simulink library "halin"  (R2021b)
settings: Solver=VariableStepAuto  StartTime=0.0  StopTime=10.0  RelTol=1e-3
undefined symbols (not defined in the file): KHAL_CAN1ABM1E2E_flg, KHAL_CAN1EPB1E2E_flg, KHAL_CAN1EPS1E2E_flg, KHAL_CAN1ESC1E2E_flg, KHAL_CAN1ESC5E2E_flg, KHAL_CAN3BMS1E2E_flg, KHAL_CAN3BMS6E2E_flg, KHAL_CAN3CCU1E2E_flg, KHAL_CAN3CCU2E2E_flg, KHAL_CAN3MCUNF1E2E_flg, KHAL_CAN3MCUNR1E2E_flg, KHAL_CAN3Shifter1E2E_flg, KHAL_CAN3Shifter2E2E_flg, KHAL_CAN6FCM2E2E_flg, KHAL_CAN6FCM4E2E_flg, TRUE
libraries: simulink x645, FVT_lib x207, hcu_lib x59
(part 22 of 23)

== system halin/HAL_IN/CAN4/ZONE_FR_VCU/SOV2Err ==
  SOV2_Err : Inport
  UnitConverter : DataTypeConversion  OutDataTypeStr=uint8
  VHAL_SOV2Err_enum : Outport
  wires:
  UnitConverter/1 -> VHAL_SOV2Err_enum/1
  SOV2_Err/1 -> UnitConverter/1

== system halin/HAL_IN/CAN4/ZONE_FR_VCU/SOV3Err ==
  SOV3_Err : Inport
  UnitConverter : DataTypeConversion  OutDataTypeStr=uint8
  VHAL_SOV3Err_enum : Outport
  wires:
  UnitConverter/1 -> VHAL_SOV3Err_enum/1
  SOV3_Err/1 -> UnitConverter/1

== system halin/HAL_IN/CAN4/ZONE_FR_VCU/Tamb ==
  Tamb : Inport
  UnitConverter : DataTypeConversion  OutDataTypeStr=uint8
  convert_in : FVT_lib/hal/convert_in  gain=0.5  offset=-40
  VHAL_Tamb_C : Outport
  wires:
  convert_in/1 -> VHAL_Tamb_C/1
  UnitConverter/1 -> convert_in/1
  Tamb/1 -> UnitConverter/1

== system halin/HAL_IN/CAN4/ZONE_FR_VCU/TambErr ==
  Tamb_Err : Inport
  UnitConverter : DataTypeConversion  OutDataTypeStr=uint8
  VHAL_TambErr_enum : Outport
  wires:
  UnitConverter/1 -> VHAL_TambErr_enum/1
  Tamb_Err/1 -> UnitConverter/1

== system halin/HAL_IN/CAN4/zGW_APTC1/FrntPTCLeActHeatPwr ==
  FrntPTCLeActHeatPwr : Inport
  UnitConverter : DataTypeConversion  OutDataTypeStr=uint8
  convert_in : FVT_lib/hal/convert_in  gain=25  offset=0
  VHAL_FrntPTCLeActHeatPwr_W : Outport
  wires:
  convert_in/1 -> VHAL_FrntPTCLeActHeatPwr_W/1
  UnitConverter/1 -> convert_in/1
  FrntPTCLeActHeatPwr/1 -> UnitConverter/1

== system halin/HAL_IN/CAN4/zGW_APTC1/FrntPTCRearLeActHeatPwr ==
  FrntPTCRearLeActHeatPwr : Inport
  UnitConverter : DataTypeConversion  OutDataTypeStr=uint8
  convert_in : FVT_lib/hal/convert_in  gain=25  offset=0
  VHAL_FrntPTCRearLeActHeatPwr_W : Outport
  wires:
  convert_in/1 -> VHAL_FrntPTCRearLeActHeatPwr_W/1
  UnitConverter/1 -> convert_in/1
  FrntPTCRearLeActHeatPwr/1 -> UnitConverter/1

== system halin/HAL_IN/CAN4/zGW_APTC1/FrntPTCRearRiActHeatPwr ==
  FrntPTCRearRiActHeatPwr : Inport
  UnitConverter : DataTypeConversion  OutDataTypeStr=uint8
  convert_in : FVT_lib/hal/convert_in  gain=25  offset=0
  VHAL_FrntPTCRearRiActHeatPwr_W : Outport
  wires:
  convert_in/1 -> VHAL_FrntPTCRearRiActHeatPwr_W/1
  UnitConverter/1 -> convert_in/1
  FrntPTCRearRiActHeatPwr/1 -> UnitConverter/1

== system halin/HAL_IN/CAN4/zGW_APTC1/FrntPTCRiActHeatPwr ==
  FrntPTCRiActHeatPwr : Inport
  UnitConverter : DataTypeConversion  OutDataTypeStr=uint8
  convert_in : FVT_lib/hal/convert_in  gain=25  offset=0
  VHAL_FrntPTCRiActHeatPwr_W : Outport
  wires:
  convert_in/1 -> VHAL_FrntPTCRiActHeatPwr_W/1
  UnitConverter/1 -> convert_in/1
  FrntPTCRiActHeatPwr/1 -> UnitConverter/1

== system halin/HAL_IN/CAN4/zGW_CANFr1/COMPActualPwr ==
  COMP_ActualPwr : Inport
  UnitConverter : DataTypeConversion  OutDataTypeStr=uint16
  VHAL_COMPActualPwr_W : Outport
  wires:
  UnitConverter/1 -> VHAL_COMPActualPwr_W/1
  COMP_ActualPwr/1 -> UnitConverter/1

== system halin/HAL_IN/CAN4/zGW_CANFr1/COMPConCur ==
  COMP_ConCur : Inport
  UnitConverter : DataTypeConversion  OutDataTypeStr=uint16
  convert_in : FVT_lib/hal/convert_in  gain=0.02  offset=0
  VHAL_COMPConCur_A : Outport
  wires:
  convert_in/1 -> VHAL_COMPConCur_A/1
  UnitConverter/1 -> convert_in/1
  COMP_ConCur/1 -> UnitConverter/1

== system halin/HAL_IN/CAN4/zGW_CANFr1/COMPConVolt ==
  COMP_ConVolt : Inport
  UnitConverter : DataTypeConversion  OutDataTypeStr=uint16
  convert_in : FVT_lib/hal/convert_in  gain=0.02  offset=0
  VHAL_COMPConVolt_V : Outport
  wires:
  convert_in/1 -> VHAL_COMPConVolt_V/1
  UnitConverter/1 -> convert_in/1
  COMP_ConVolt/1 -> UnitConverter/1

== system halin/HAL_IN/CAN4/zGW_CANFr1/COMPStatorSpd ==
  COMP_StatorSpd : Inport
  UnitConverter : DataTypeConversion  OutDataTypeStr=uint16
  VHAL_COMPStatorSpd_rpm : Outport
  wires:
  UnitConverter/1 -> VHAL_COMPStatorSpd_rpm/1
  COMP_StatorSpd/1 -> UnitConverter/1

== system halin/HAL_IN/CAN4/zGW_CANFr1/PTC1PowerConsumption ==
  PTC1_PowerConsumption : Inport
  UnitConverter : DataTypeConversion  OutDataTypeStr=uint8
  convert_in : FVT_lib/hal/convert_in  gain=0.1  offset=0
  VHAL_PTC1PowerConsumption_kW : Outport
  wires:
  convert_in/1 -> VHAL_PTC1PowerConsumption_kW/1
  UnitConverter/1 -> convert_in/1
  PTC1_PowerConsumption/1 -> UnitConverter/1

== system halin/HAL_IN/CAN4/zGW_LINDr1/CSWDimSw ==
  CSW_DimSw : Inport
  UnitConverter : DataTypeConversion  OutDataTypeStr=uint8
  VHAL_CSWDimSw_flg : Outport
  wires:
  UnitConverter/1 -> VHAL_CSWDimSw_flg/1
  CSW_DimSw/1 -> UnitConverter/1

== system halin/HAL_IN/CAN4/zGW_LINDr1/CSWFWasSwSta ==
  CSW_FWasSw_Sta : Inport
  UnitConverter : DataTypeConversion  OutDataTypeStr=uint8
  VHAL_CSWFWasSwSta_enum : Outport
  wires:
  UnitConverter/1 -> VHAL_CSWFWasSwSta_enum/1
  CSW_FWasSw_Sta/1 -> UnitConverter/1

== system halin/HAL_IN/CAN4/zGW_LINDr1/CSWFWipSwSta ==
  CSW_FWipSw_Sta : Inport
  UnitConverter : DataTypeConversion  OutDataTypeStr=uint8
  VHAL_CSWFWipSwSta_enum : Outport
  wires:
  UnitConverter/1 -> VHAL_CSWFWipSwSta_enum/1
  CSW_FWipSw_Sta/1 -> UnitConverter/1

== system halin/HAL_IN/CAN4/zGW_LINDr1/CSWPassSWSta ==
  CSW_PassSW_Sta : Inport
  UnitConverter : DataTypeConversion  OutDataTypeStr=uint8
  VHAL_CSWPassSWSta_flg : Outport
  wires:
  UnitConverter/1 -> VHAL_CSWPassSWSta_flg/1
  CSW_PassSW_Sta/1 -> UnitConverter/1

== system halin/HAL_IN/CAN4/zGW_LINDr1/CSWRWasSWSta ==
  CSW_RWasSW_Sta : Inport
  UnitConverter : DataTypeConversion  OutDataTypeStr=uint8
  VHAL_CSWRWasSWSta_enum : Outport
  wires:
  UnitConverter/1 -> VHAL_CSWRWasSWSta_enum/1
  CSW_RWasSW_Sta/1 -> UnitConverter/1

== system halin/HAL_IN/CAN4/zGW_LINDr1/CSWRWipIntSwSta ==
  CSW_RWipIntSw_Sta : Inport
  UnitConverter : DataTypeConversion  OutDataTypeStr=uint8
  VHAL_CSWRWipIntSwSta_enum : Outport
  wires:
  UnitConverter/1 -> VHAL_CSWRWipIntSwSta_enum/1
  CSW_RWipIntSw_Sta/1 -> UnitConverter/1

== system halin/HAL_IN/CAN4/zGW_LINDr1/CSWTurnSwSta ==
  CSW_TurnSw_Sta : Inport
  UnitConverter : DataTypeConversion  OutDataTypeStr=uint8
  VHAL_CSWTurnSwSta_enum : Outport
  wires:
  UnitConverter/1 -> VHAL_CSWTurnSwSta_enum/1
  CSW_TurnSw_Sta/1 -> UnitConverter/1

== system halin/HAL_IN/CAN4/zGW_LINDr1/FAPWL01LINResponseError ==
  FAPWL_01_LIN_Response_Error : Inport
  UnitConverter : DataTypeConversion  OutDataTypeStr=uint8
  VHAL_FAPWL01LINResponseError_flg : Outport
  wires:
  UnitConverter/1 -> VHAL_FAPWL01LINResponseError_flg/1
  FAPWL_01_LIN_Response_Error/1 -> UnitConverter/1

== system halin/HAL_IN/CAN4/zGW_LINDr1/LDrvMotorRelayError ==
  L_Drv_Motor_Relay_Error : Inport
  UnitConverter : DataTypeConversion  OutDataTypeStr=uint8
  VHAL_LDrvMotorRelayError_flg : Outport
  wires:
  UnitConverter/1 -> VHAL_LDrvMotorRelayError_flg/1
  L_Drv_Motor_Relay_Error/1 -> UnitConverter/1

== system halin/HAL_IN/CAN4/zGW_LINDr1/LDrvMotorRippleError ==
  L_Drv_Motor_Ripple_Error : Inport
  UnitConverter : DataTypeConversion  OutDataTypeStr=uint8
  VHAL_LDrvMotorRippleError_flg : Outport
  wires:
  UnitConverter/1 -> VHAL_LDrvMotorRippleError_flg/1
  L_Drv_Motor_Ripple_Error/1 -> UnitConverter/1

== system halin/HAL_IN/CAN4/zGW_LINDr1/LDrvValWdwOpened ==
  L_Drv_Val_Wdw_Opened : Inport
  UnitConverter : DataTypeConversion  OutDataTypeStr=uint8
  VHAL_LDrvValWdwOpened_pct : Outport
  wires:
  UnitConverter/1 -> VHAL_LDrvValWdwOpened_pct/1
  L_Drv_Val_Wdw_Opened/1 -> UnitConverter/1

== system halin/HAL_IN/CAN4/zGW_LINDr1/LDrvWdwPositionSts ==
  L_Drv_Wdw_PositionSts : Inport
  UnitConverter : DataTypeConversion  OutDataTypeStr=uint8
  VHAL_LDrvWdwPositionSts_enum : Outport
  wires:
  UnitConverter/1 -> VHAL_LDrvWdwPositionSts_enum/1
  L_Drv_Wdw_PositionSts/1 -> UnitConverter/1

== system halin/HAL_IN/CAN4/zGW_LINDr1/LPasMotorRelayError ==
  L_Pas_Motor_Relay_Error : Inport
  UnitConverter : DataTypeConversion  OutDataTypeStr=uint8
  VHAL_LPasMotorRelayError_flg : Outport
  wires:
  UnitConverter/1 -> VHAL_LPasMotorRelayError_flg/1
  L_Pas_Motor_Relay_Error/1 -> UnitConverter/1

== system halin/HAL_IN/CAN4/zGW_LINDr1/LPasMotorRippleError ==
  L_Pas_Motor_Ripple_Error : Inport
  UnitConverter : DataTypeConversion  OutDataTypeStr=uint8
  VHAL_LPasMotorRippleError_flg : Outport
  wires:
  UnitConverter/1 -> VHAL_LPasMotorRippleError_flg/1
  L_Pas_Motor_Ripple_Error/1 -> UnitConverter/1

== system halin/HAL_IN/CAN4/zGW_LINDr1/LPasValWdwOpened ==
  L_Pas_Val_Wdw_Opened : Inport
  UnitConverter : DataTypeConversion  OutDataTypeStr=uint8
  VHAL_LPasValWdwOpened_pct : Outport
  wires:
  UnitConverter/1 -> VHAL_LPasValWdwOpened_pct/1
  L_Pas_Val_Wdw_Opened/1 -> UnitConverter/1

== system halin/HAL_IN/CAN4/zGW_LINDr1/LPasWdwPositionSts ==
  L_Pas_Wdw_PositionSts : Inport
  UnitConverter : DataTypeConversion  OutDataTypeStr=uint8
  VHAL_LPasWdwPositionSts_enum : Outport
  wires:
  UnitConverter/1 -> VHAL_LPasWdwPositionSts_enum/1
  L_Pas_Wdw_PositionSts/1 -> UnitConverter/1

== system halin/HAL_IN/CAN4/zGW_LINDr1/LRLDMotorRelayError ==
  L_RLD_Motor_Relay_Error : Inport
  UnitConverter : DataTypeConversion  OutDataTypeStr=uint8
  VHAL_LRLDMotorRelayError_flg : Outport
  wires:
  UnitConverter/1 -> VHAL_LRLDMotorRelayError_flg/1
  L_RLD_Motor_Relay_Error/1 -> UnitConverter/1

== system halin/HAL_IN/CAN4/zGW_LINDr1/LRLDMotorRippleError ==
  L_RLD_Motor_Ripple_Error : Inport
  UnitConverter : DataTypeConversion  OutDataTypeStr=uint8
  VHAL_LRLDMotorRippleError_flg : Outport
  wires:
  UnitConverter/1 -> VHAL_LRLDMotorRippleError_flg/1
  L_RLD_Motor_Ripple_Error/1 -> UnitConverter/1

== system halin/HAL_IN/CAN4/zGW_LINDr1/LRLDValWdwOpened ==
  L_RLD_Val_Wdw_Opened : Inport
  UnitConverter : DataTypeConversion  OutDataTypeStr=uint8
  VHAL_LRLDValWdwOpened_pct : Outport
  wires:
  UnitConverter/1 -> VHAL_LRLDValWdwOpened_pct/1
  L_RLD_Val_Wdw_Opened/1 -> UnitConverter/1

== system halin/HAL_IN/CAN4/zGW_LINDr1/LRLDWdwPositionSts ==
  L_RLD_Wdw_PositionSts : Inport
  UnitConverter : DataTypeConversion  OutDataTypeStr=uint8
  VHAL_LRLDWdwPositionSts_enum : Outport
  wires:
  UnitConverter/1 -> VHAL_LRLDWdwPositionSts_enum/1
  L_RLD_Wdw_PositionSts/1 -> UnitConverter/1

== system halin/HAL_IN/CAN4/zGW_LINDr1/LRRDMotorRelayError ==
  L_RRD_Motor_Relay_Error : Inport
  UnitConverter : DataTypeConversion  OutDataTypeStr=uint8
  VHAL_LRRDMotorRelayError_flg : Outport
  wires:
  UnitConverter/1 -> VHAL_LRRDMotorRelayError_flg/1
  L_RRD_Motor_Relay_Error/1 -> UnitConverter/1

== system halin/HAL_IN/CAN4/zGW_LINDr1/LRRDMotorRippleError ==
  L_RRD_Motor_Ripple_Error : Inport
  UnitConverter : DataTypeConversion  OutDataTypeStr=uint8
  VHAL_LRRDMotorRippleError_flg : Outport
  wires:
  UnitConverter/1 -> VHAL_LRRDMotorRippleError_flg/1
  L_RRD_Motor_Ripple_Error/1 -> UnitConverter/1

== system halin/HAL_IN/CAN4/zGW_LINDr1/LRRDValWdwOpened ==
  L_RRD_Val_Wdw_Opened : Inport
  UnitConverter : DataTypeConversion  OutDataTypeStr=uint8
  VHAL_LRRDValWdwOpened_pct : Outport
  wires:
  UnitConverter/1 -> VHAL_LRRDValWdwOpened_pct/1
  L_RRD_Val_Wdw_Opened/1 -> UnitConverter/1

== system halin/HAL_IN/CAN4/zGW_LINDr1/LRRDWdwPositionSts ==
  L_RRD_Wdw_PositionSts : Inport
  UnitConverter : DataTypeConversion  OutDataTypeStr=uint8
  VHAL_LRRDWdwPositionSts_enum : Outport
  wires:
  UnitConverter/1 -> VHAL_LRRDWdwPositionSts_enum/1
  L_RRD_Wdw_PositionSts/1 -> UnitConverter/1

== system halin/HAL_IN/CAN4/zGW_LINDr1/RAPWL01LINResponseError ==
  RAPWL_01_LIN_Response_Error : Inport
  UnitConverter : DataTypeConversion  OutDataTypeStr=uint8
  VHAL_RAPWL01LINResponseError_flg : Outport
  wires:
  UnitConverter/1 -> VHAL_RAPWL01LINResponseError_flg/1
  RAPWL_01_LIN_Response_Error/1 -> UnitConverter/1

== system halin/HAL_IN/CAN4/zGW_LINDr1/RLSLampSta ==
  RLS_Lamp_Sta : Inport
  UnitConverter : DataTypeConversion  OutDataTypeStr=uint8
  VHAL_RLSLampSta_flg : Outport
  wires:
  UnitConverter/1 -> VHAL_RLSLampSta_flg/1
  RLS_Lamp_Sta/1 -> UnitConverter/1

== system halin/HAL_IN/CAN4/zGW_LINDr1/RLSRainSnrWiperCmd ==
  RLS_RainSnrWiperCmd : Inport
  UnitConverter : DataTypeConversion  OutDataTypeStr=uint8
  VHAL_RLSRainSnrWiperCmd_enum : Outport
  wires:
  UnitConverter/1 -> VHAL_RLSRainSnrWiperCmd_enum/1
  RLS_RainSnrWiperCmd/1 -> UnitConverter/1

== system halin/HAL_IN/CAN4/zGW_LINDr1/SWC2LADASSta ==
  SWC2_L_ADAS_Sta : Inport
  UnitConverter : DataTypeConversion  OutDataTypeStr=uint8
  VHAL_SWC2LADASSta_flg : Outport
  wires:
  UnitConverter/1 -> VHAL_SWC2LADASSta_flg/1
  SWC2_L_ADAS_Sta/1 -> UnitConverter/1

== system halin/HAL_IN/CAN4/zGW_LINDr1/SWC2LDriveModeSta ==
  SWC2_L_DriveMode_Sta : Inport
  UnitConverter : DataTypeConversion  OutDataTypeStr=uint8
  VHAL_SWC2LDriveModeSta_flg : Outport
  wires:
  UnitConverter/1 -> VHAL_SWC2LDriveModeSta_flg/1
  SWC2_L_DriveMode_Sta/1 -> UnitConverter/1

== system halin/HAL_IN/CAN4/zGW_LINDr1/SWC2LHomeSta ==
  SWC2_L_Home_Sta : Inport
  UnitConverter : DataTypeConversion  OutDataTypeStr=uint8
  VHAL_SWC2LHomeSta_flg : Outport
  wires:
  UnitConverter/1 -> VHAL_SWC2LHomeSta_flg/1
  SWC2_L_Home_Sta/1 -> UnitConverter/1

== system halin/HAL_IN/CAN4/zGW_LINDr1/SWC2LLeftSta ==
  SWC2_L_Left_Sta : Inport
  UnitConverter : DataTypeConversion  OutDataTypeStr=uint8
  VHAL_SWC2LLeftSta_flg : Outport
  wires:
  UnitConverter/1 -> VHAL_SWC2LLeftSta_flg/1
  SWC2_L_Left_Sta/1 -> UnitConverter/1

== system halin/HAL_IN/CAN4/zGW_LINDr1/SWC2LRegenUpSta ==
  SWC2_L_RegenUp_Sta : Inport
  UnitConverter : DataTypeConversion  OutDataTypeStr=uint8
  VHAL_SWC2LRegenUpSta_flg : Outport
  wires:
  UnitConverter/1 -> VHAL_SWC2LRegenUpSta_flg/1
  SWC2_L_RegenUp_Sta/1 -> UnitConverter/1

== system halin/HAL_IN/CAN4/zGW_LINDr1/SWC2LRightSta ==
  SWC2_L_Right_Sta : Inport
  UnitConverter : DataTypeConversion  OutDataTypeStr=uint8
  VHAL_SWC2LRightSta_flg : Outport
  wires:
  UnitConverter/1 -> VHAL_SWC2LRightSta_flg/1
  SWC2_L_Right_Sta/1 -> UnitConverter/1

== system halin/HAL_IN/CAN4/zGW_LINDr1/SWC2LScrollDownSta ==
  SWC2_L_ScrollDown_Sta : Inport
  UnitConverter : DataTypeConversion  OutDataTypeStr=uint8
  VHAL_SWC2LScrollDownSta_flg : Outport
  wires:
  UnitConverter/1 -> VHAL_SWC2LScrollDownSta_flg/1
  SWC2_L_ScrollDown_Sta/1 -> UnitConverter/1

== system halin/HAL_IN/CAN4/zGW_LINDr1/SWC2LScrollPressSta ==
  SWC2_L_ScrollPress_Sta : Inport
  UnitConverter : DataTypeConversion  OutDataTypeStr=uint8
  VHAL_SWC2LScrollPressSta_flg : Outport
  wires:
  UnitConverter/1 -> VHAL_SWC2LScrollPressSta_flg/1
  SWC2_L_ScrollPress_Sta/1 -> UnitConverter/1

== system halin/HAL_IN/CAN4/zGW_LINDr1/SWC2LScrollUpSta ==
  SWC2_L_ScrollUp_Sta : Inport
  UnitConverter : DataTypeConversion  OutDataTypeStr=uint8
  VHAL_SWC2LScrollUpSta_flg : Outport
  wires:
  UnitConverter/1 -> VHAL_SWC2LScrollUpSta_flg/1
  SWC2_L_ScrollUp_Sta/1 -> UnitConverter/1

== system halin/HAL_IN/CAN4/zGW_LINDr1/SWC2RCustomizeSta ==
  SWC2_R_Customize_Sta : Inport
  UnitConverter : DataTypeConversion  OutDataTypeStr=uint8
  VHAL_SWC2RCustomizeSta_flg : Outport
  wires:
  UnitConverter/1 -> VHAL_SWC2RCustomizeSta_flg/1
  SWC2_R_Customize_Sta/1 -> UnitConverter/1

== system halin/HAL_IN/CAN4/zGW_LINDr1/SWC2RLeftSta ==
  SWC2_R_Left_Sta : Inport
  UnitConverter : DataTypeConversion  OutDataTypeStr=uint8
  VHAL_SWC2RLeftSta_flg : Outport
  wires:
  UnitConverter/1 -> VHAL_SWC2RLeftSta_flg/1
  SWC2_R_Left_Sta/1 -> UnitConverter/1

== system halin/HAL_IN/CAN4/zGW_LINDr1/SWC2RPageSwitchSta ==
  SWC2_R_PageSwitch_Sta : Inport
  UnitConverter : DataTypeConversion  OutDataTypeStr=uint8
  VHAL_SWC2RPageSwitchSta_flg : Outport
  wires:
  UnitConverter/1 -> VHAL_SWC2RPageSwitchSta_flg/1
  SWC2_R_PageSwitch_Sta/1 -> UnitConverter/1

== system halin/HAL_IN/CAN4/zGW_LINDr1/SWC2RRegenDownSta ==
  SWC2_R_RegenDown_Sta : Inport
  UnitConverter : DataTypeConversion  OutDataTypeStr=uint8
  VHAL_SWC2RRegenDownSta_flg : Outport
  wires:
  UnitConverter/1 -> VHAL_SWC2RRegenDownSta_flg/1
  SWC2_R_RegenDown_Sta/1 -> UnitConverter/1

== system halin/HAL_IN/CAN4/zGW_LINDr1/SWC2RRightSta ==
  SWC2_R_Right_Sta : Inport
  UnitConverter : DataTypeConversion  OutDataTypeStr=uint8
  VHAL_SWC2RRightSta_flg : Outport
  wires:
  UnitConverter/1 -> VHAL_SWC2RRightSta_flg/1
  SWC2_R_Right_Sta/1 -> UnitConverter/1

== system halin/HAL_IN/CAN4/zGW_LINDr1/SWC2RScrollDownSta ==
  SWC2_R_ScrollDown_Sta : Inport
  UnitConverter : DataTypeConversion  OutDataTypeStr=uint8
  VHAL_SWC2RScrollDownSta_flg : Outport
  wires:
  UnitConverter/1 -> VHAL_SWC2RScrollDownSta_flg/1
  SWC2_R_ScrollDown_Sta/1 -> UnitConverter/1

== system halin/HAL_IN/CAN4/zGW_LINDr1/SWC2RScrollPressSta ==
  SWC2_R_ScrollPress_Sta : Inport
  UnitConverter : DataTypeConversion  OutDataTypeStr=uint8
  VHAL_SWC2RScrollPressSta_flg : Outport
  wires:
  UnitConverter/1 -> VHAL_SWC2RScrollPressSta_flg/1
  SWC2_R_ScrollPress_Sta/1 -> UnitConverter/1

== system halin/HAL_IN/CAN4/zGW_LINDr1/SWC2RScrollUpSta ==
  SWC2_R_ScrollUp_Sta : Inport
  UnitConverter : DataTypeConversion  OutDataTypeStr=uint8
  VHAL_SWC2RScrollUpSta_flg : Outport
  wires:
  UnitConverter/1 -> VHAL_SWC2RScrollUpSta_flg/1
  SWC2_R_ScrollUp_Sta/1 -> UnitConverter/1

== system halin/HAL_IN/CAN4/zGW_LINDr1/SWC2RVRSta ==
  SWC2_R_VR_Sta : Inport
  UnitConverter : DataTypeConversion  OutDataTypeStr=uint8
  VHAL_SWC2RVRSta_flg : Outport
  wires:
  UnitConverter/1 -> VHAL_SWC2RVRSta_flg/1
  SWC2_R_VR_Sta/1 -> UnitConverter/1

== system halin/HAL_IN/CAN4/zGW_LINDr1/SWCACCSta ==
  SWC_ACC_Sta : Inport
  UnitConverter : DataTypeConversion  OutDataTypeStr=uint8
  VHAL_SWCACCSta_flg : Outport
  wires:
  UnitConverter/1 -> VHAL_SWCACCSta_flg/1
  SWC_ACC_Sta/1 -> UnitConverter/1

== system halin/HAL_IN/CAN4/zGW_LINDr1/SWCCANCELSta ==
  SWC_CANCEL_Sta : Inport
  UnitConverter : DataTypeConversion  OutDataTypeStr=uint8
  VHAL_SWCCANCELSta_flg : Outport
  wires:
  UnitConverter/1 -> VHAL_SWCCANCELSta_flg/1
  SWC_CANCEL_Sta/1 -> UnitConverter/1

== system halin/HAL_IN/CAN4/zGW_LINDr1/SWCDistanceSta ==
  SWC_Distance_Sta : Inport
  UnitConverter : DataTypeConversion  OutDataTypeStr=uint8
  VHAL_SWCDistanceSta_flg : Outport
  wires:
  UnitConverter/1 -> VHAL_SWCDistanceSta_flg/1
  SWC_Distance_Sta/1 -> UnitConverter/1

== system halin/HAL_IN/CAN4/zGW_LINDr1/SWCDownSta ==
  SWC_Down_Sta : Inport
  UnitConverter : DataTypeConversion  OutDataTypeStr=uint8
  VHAL_SWCDownSta_flg : Outport
  wires:
  UnitConverter/1 -> VHAL_SWCDownSta_flg/1
  SWC_Down_Sta/1 -> UnitConverter/1

== system halin/HAL_IN/CAN4/zGW_LINDr1/SWCLKASta ==
  SWC_LKA_Sta : Inport
  UnitConverter : DataTypeConversion  OutDataTypeStr=uint8
  VHAL_SWCLKASta_flg : Outport
  wires:
  UnitConverter/1 -> VHAL_SWCLKASta_flg/1
  SWC_LKA_Sta/1 -> UnitConverter/1

== system halin/HAL_IN/CAN4/zGW_LINDr1/SWCLeftSta ==
  SWC_Left_Sta : Inport
  UnitConverter : DataTypeConversion  OutDataTypeStr=uint8
  VHAL_SWCLeftSta_flg : Outport
  wires:
  UnitConverter/1 -> VHAL_SWCLeftSta_flg/1
  SWC_Left_Sta/1 -> UnitConverter/1

== system halin/HAL_IN/CAN4/zGW_LINDr1/SWCRegenDown ==
  SWC_RegenDown : Inport
  UnitConverter : DataTypeConversion  OutDataTypeStr=uint8
  VHAL_SWCRegenDown_flg : Outport
  wires:
  UnitConverter/1 -> VHAL_SWCRegenDown_flg/1
  SWC_RegenDown/1 -> UnitConverter/1

== system halin/HAL_IN/CAN4/zGW_LINDr1/SWCRegenUp ==
  SWC_RegenUp : Inport
  UnitConverter : DataTypeConversion  OutDataTypeStr=uint8
  VHAL_SWCRegenUp_flg : Outport
  wires:
  UnitConverter/1 -> VHAL_SWCRegenUp_flg/1
  SWC_RegenUp/1 -> UnitConverter/1

== system halin/HAL_IN/CAN4/zGW_LINDr1/SWCResUpSta ==
  SWC_Res_Up_Sta : Inport
  UnitConverter : DataTypeConversion  OutDataTypeStr=uint8
  VHAL_SWCResUpSta_flg : Outport
  wires:
  UnitConverter/1 -> VHAL_SWCResUpSta_flg/1
  SWC_Res_Up_Sta/1 -> UnitConverter/1

== system halin/HAL_IN/CAN4/zGW_LINDr1/SWCRightSta ==
  SWC_Right_Sta : Inport
  UnitConverter : DataTypeConversion  OutDataTypeStr=uint8
  VHAL_SWCRightSta_flg : Outport
  wires:
  UnitConverter/1 -> VHAL_SWCRightSta_flg/1
  SWC_Right_Sta/1 -> UnitConverter/1

== system halin/HAL_IN/CAN4/zGW_LINDr1/SWCSetdownSta ==
  SWC_Set_down_Sta : Inport
  UnitConverter : DataTypeConversion  OutDataTypeStr=uint8
  VHAL_SWCSetdownSta_flg : Outport
  wires:
  UnitConverter/1 -> VHAL_SWCSetdownSta_flg/1
  SWC_Set_down_Sta/1 -> UnitConverter/1

== system halin/HAL_IN/CAN4/zGW_LINDr1/SWCTripSta ==
  SWC_Trip_Sta : Inport
  UnitConverter : DataTypeConversion  OutDataTypeStr=uint8
  VHAL_SWCTripSta_flg : Outport
  wires:
  UnitConverter/1 -> VHAL_SWCTripSta_flg/1
  SWC_Trip_Sta/1 -> UnitConverter/1

== system halin/HAL_IN/CAN4/zGW_LINDr1/SWCUndefinedSta ==
  SWC_Undefined_Sta : Inport
  UnitConverter : DataTypeConversion  OutDataTypeStr=uint8
  VHAL_SWCUndefinedSta_flg : Outport
  wires:
  UnitConverter/1 -> VHAL_SWCUndefinedSta_flg/1
  SWC_Undefined_Sta/1 -> UnitConverter/1

== system halin/HAL_IN/CAN4/zGW_LINDr1/SWCUpSta ==
  SWC_Up_Sta : Inport
  UnitConverter : DataTypeConversion  OutDataTypeStr=uint8
  VHAL_SWCUpSta_flg : Outport
  wires:
  UnitConverter/1 -> VHAL_SWCUpSta_flg/1
  SWC_Up_Sta/1 -> UnitConverter/1

== system halin/HAL_IN/CAN4/zGW_LINDr1/SWCVRSta ==
  SWC_VR_Sta : Inport
  UnitConverter : DataTypeConversion  OutDataTypeStr=uint8
  VHAL_SWCVRSta_flg : Outport
  wires:
  UnitConverter/1 -> VHAL_SWCVRSta_flg/1
  SWC_VR_Sta/1 -> UnitConverter/1

== system halin/HAL_IN/CAN4/zGW_LINDr1/SWCmodeSta ==
  SWC_mode_Sta : Inport
  UnitConverter : DataTypeConversion  OutDataTypeStr=uint8
  VHAL_SWCmodeSta_flg : Outport
  wires:
  UnitConverter/1 -> VHAL_SWCmodeSta_flg/1
  SWC_mode_Sta/1 -> UnitConverter/1

== system halin/HAL_IN/CAN4/zGW_LINDr2/ACT1ResponseError ==
  ACT1_Response_Error : Inport
  UnitConverter : DataTypeConversion  OutDataTypeStr=uint8
  VHAL_ACT1ResponseError_flg : Outport
  wires:
  UnitConverter/1 -> VHAL_ACT1ResponseError_flg/1
  ACT1_Response_Error/1 -> UnitConverter/1

== system halin/HAL_IN/CAN4/zGW_LINFr1/AGSActualPosition ==
  AGS_Actual_Position : Inport
  UnitConverter : DataTypeConversion  OutDataTypeStr=uint8
  VHAL_AGSActualPosition_enum : Outport
  wires:
  UnitConverter/1 -> VHAL_AGSActualPosition_enum/1
  AGS_Actual_Position/1 -> UnitConverter/1

== system halin/HAL_IN/CAN4/zGW_LINFr1/FGSIntenRspSta ==
  FGS_IntenRsp_Sta : Inport
  UnitConverter : DataTypeConversion  OutDataTypeStr=uint8
  VHAL_FGSIntenRspSta_enum : Outport
  wires:
  UnitConverter/1 -> VHAL_FGSIntenRspSta_enum/1
  FGS_IntenRsp_Sta/1 -> UnitConverter/1

== system halin/HAL_IN/CAN4/zGW_LINFr2/EWP1BlockError ==
  EWP1_Block_Error : Inport
  UnitConverter : DataTypeConversion  OutDataTypeStr=uint8
  VHAL_EWP1BlockError_enum : Outport
  wires:
  UnitConverter/1 -> VHAL_EWP1BlockError_enum/1
  EWP1_Block_Error/1 -> UnitConverter/1

== system halin/HAL_IN/CAN4/zGW_LINFr2/EWP1OverCurrError ==
  EWP1_OverCurr_Error : Inport
  UnitConverter : DataTypeConversion  OutDataTypeStr=uint8
  VHAL_EWP1OverCurrError_enum : Outport
  wires:
  UnitConverter/1 -> VHAL_EWP1OverCurrError_enum/1
  EWP1_OverCurr_Error/1 -> UnitConverter/1

== system halin/HAL_IN/CAN4/zGW_LINFr2/EWP2BlockError ==
  EWP2_Block_Error : Inport
  UnitConverter : DataTypeConversion  OutDataTypeStr=uint8
  VHAL_EWP2BlockError_enum : Outport
  wires:
  UnitConverter/1 -> VHAL_EWP2BlockError_enum/1
  EWP2_Block_Error/1 -> UnitConverter/1

== system halin/HAL_IN/CAN4/zGW_LINFr2/EWP2OverCurrError ==
  EWP2_OverCurr_Error : Inport
  UnitConverter : DataTypeConversion  OutDataTypeStr=uint8
  VHAL_EWP2OverCurrError_enum : Outport
  wires:
  UnitConverter/1 -> VHAL_EWP2OverCurrError_enum/1
  EWP2_OverCurr_Error/1 -> UnitConverter/1

== system halin/HAL_IN/CAN4/zGW_LINFr2/EWP3BlockError ==
  EWP3_Block_Error : Inport
  UnitConverter : DataTypeConversion  OutDataTypeStr=uint8
  VHAL_EWP3BlockError_enum : Outport
  wires:
  UnitConverter/1 -> VHAL_EWP3BlockError_enum/1
  EWP3_Block_Error/1 -> UnitConverter/1

== system halin/HAL_IN/CAN4/zGW_LINFr2/EWP3OverCurrError ==
  EWP3_OverCurr_Error : Inport
  UnitConverter : DataTypeConversion  OutDataTypeStr=uint8
  VHAL_EWP3OverCurrError_enum : Outport
  wires:
  UnitConverter/1 -> VHAL_EWP3OverCurrError_enum/1
  EWP3_OverCurr_Error/1 -> UnitConverter/1

== system halin/HAL_IN/CAN4/zGW_SEAT1/DSEATAntiSta ==
  DSEAT_Anti_Sta : Inport
  UnitConverter : DataTypeConversion  OutDataTypeStr=uint8
  VHAL_DSEATAntiSta_flg : Outport
  wires:
  UnitConverter/1 -> VHAL_DSEATAntiSta_flg/1
  DSEAT_Anti_Sta/1 -> UnitConverter/1

== system halin/HAL_IN/CAN4/zGW_SEAT1/DSEATEntryFunSta ==
  DSEAT_EntryFun_Sta : Inport
  UnitConverter : DataTypeConversion  OutDataTypeStr=uint8
  VHAL_DSEATEntryFunSta_flg : Outport
  wires:
  UnitConverter/1 -> VHAL_DSEATEntryFunSta_flg/1
  DSEAT_EntryFun_Sta/1 -> UnitConverter/1

== system halin/HAL_IN/CAN4/zGW_SEAT1/DSEATErrorSta ==
  DSEAT_Error_Sta : Inport
  UnitConverter : DataTypeConversion  OutDataTypeStr=uint8
  VHAL_DSEATErrorSta_flg : Outport
  wires:
  UnitConverter/1 -> VHAL_DSEATErrorSta_flg/1
  DSEAT_Error_Sta/1 -> UnitConverter/1

== system halin/HAL_IN/CAN4/zGW_SEAT1/DSEATHWVer ==
  DSEAT_HW_Ver : Inport
  UnitConverter : DataTypeConversion  OutDataTypeStr=uint16
  VHAL_DSEATHWVer_enum : Outport
  wires:
  UnitConverter/1 -> VHAL_DSEATHWVer_enum/1
  DSEAT_HW_Ver/1 -> UnitConverter/1

== system halin/HAL_IN/CAN4/zGW_SEAT1/DSEATMode ==
  DSEAT_Mode : Inport
  UnitConverter : DataTypeConversion  OutDataTypeStr=uint8
  VHAL_DSEATMode_enum : Outport
  wires:
  UnitConverter/1 -> VHAL_DSEATMode_enum/1
  DSEAT_Mode/1 -> UnitConverter/1

== system halin/HAL_IN/CAN4/zGW_SEAT1/DSEATSWVer ==
  DSEAT_SW_Ver : Inport
  UnitConverter : DataTypeConversion  OutDataTypeStr=uint16
  VHAL_DSEATSWVer_enum : Outport
  wires:
  UnitConverter/1 -> VHAL_DSEATSWVer_enum/1
  DSEAT_SW_Ver/1 -> UnitConverter/1

== system halin/HAL_IN/CAN4/zGW_SEAT1/DSEATVentSta ==
  DSEAT_Vent_Sta : Inport
  UnitConverter : DataTypeConversion  OutDataTypeStr=uint8
  VHAL_DSEATVentSta_enum : Outport
  wires:
  UnitConverter/1 -> VHAL_DSEATVentSta_enum/1
  DSEAT_Vent_Sta/1 -> UnitConverter/1

== system halin/HAL_IN/CAN4/zGW_SEAT1/DSEATheatersta ==
  DSEAT_heater_sta : Inport
  UnitConverter : DataTypeConversion  OutDataTypeStr=uint8
  VHAL_DSEATheatersta_enum : Outport
  wires:
  UnitConverter/1 -> VHAL_DSEATheatersta_enum/1
  DSEAT_heater_sta/1 -> UnitConverter/1

== system halin/HAL_IN/CAN4/zGW_SEAT1/PSEATErrorSta ==
  PSEAT_Error_Sta : Inport
  UnitConverter : DataTypeConversion  OutDataTypeStr=uint8
  VHAL_PSEATErrorSta_flg : Outport
  wires:
  UnitConverter/1 -> VHAL_PSEATErrorSta_flg/1
  PSEAT_Error_Sta/1 -> UnitConverter/1

== system halin/HAL_IN/CAN4/zGW_SEAT1/PSEATHWVer ==
  PSEAT_HW_Ver : Inport
  UnitConverter : DataTypeConversion  OutDataTypeStr=uint16
  VHAL_PSEATHWVer_enum : Outport
  wires:
  UnitConverter/1 -> VHAL_PSEATHWVer_enum/1
  PSEAT_HW_Ver/1 -> UnitConverter/1

== system halin/HAL_IN/CAN4/zGW_SEAT1/PSEATMode ==
  PSEAT_Mode : Inport
  UnitConverter : DataTypeConversion  OutDataTypeStr=uint8
  VHAL_PSEATMode_enum : Outport
  wires:
  UnitConverter/1 -> VHAL_PSEATMode_enum/1
  PSEAT_Mode/1 -> UnitConverter/1

== system halin/HAL_IN/CAN4/zGW_SEAT1/PSEATSWVer ==
  PSEAT_SW_Ver : Inport
  UnitConverter : DataTypeConversion  OutDataTypeStr=uint16
  VHAL_PSEATSWVer_enum : Outport
  wires:
  UnitConverter/1 -> VHAL_PSEATSWVer_enum/1
  PSEAT_SW_Ver/1 -> UnitConverter/1

== system halin/HAL_IN/CAN4/zGW_SEAT1/PSEATVentSta ==
  PSEAT_Vent_Sta : Inport
  UnitConverter : DataTypeConversion  OutDataTypeStr=uint8
  VHAL_PSEATVentSta_enum : Outport
  wires:
  UnitConverter/1 -> VHAL_PSEATVentSta_enum/1
  PSEAT_Vent_Sta/1 -> UnitConverter/1

== system halin/HAL_IN/CAN4/zGW_SEAT1/PSEATheatersta ==
  PSEAT_heater_sta : Inport
  UnitConverter : DataTypeConversion  OutDataTypeStr=uint8
  VHAL_PSEATheatersta_enum : Outport
  wires:
  UnitConverter/1 -> VHAL_PSEATheatersta_enum/1
  PSEAT_heater_sta/1 -> UnitConverter/1

== system halin/HAL_IN/CAN6/FCM1/ACCComfortBandLower ==
  ACC_ComfortBandLower : Inport
  UnitConverter : DataTypeConversion  OutDataTypeStr=uint16
  convert_in : FVT_lib/hal/convert_in  gain=0.05  offset=-15
  VHAL_ACCComfortBandLower_mps2 : Outport
  wires:
  convert_in/1 -> VHAL_ACCComfortBandLower_mps2/1
  UnitConverter/1 -> convert_in/1
  ACC_ComfortBandLower/1 -> UnitConverter/1

== system halin/HAL_IN/CAN6/FCM1/ACCComfortBandUpper ==
  ACC_ComfortBandUpper : Inport
  UnitConverter : DataTypeConversion  OutDataTypeStr=uint16
  convert_in : FVT_lib/hal/convert_in  gain=0.05  offset=-15
  VHAL_ACCComfortBandUpper_mps2 : Outport
  wires:
  convert_in/1 -> VHAL_ACCComfortBandUpper_mps2/1
  UnitConverter/1 -> convert_in/1
  ACC_ComfortBandUpper/1 -> UnitConverter/1

== system halin/HAL_IN/CAN6/FCM1/ACCJerkLowerLimit ==
  ACC_JerkLowerLimit : Inport
  UnitConverter : DataTypeConversion  OutDataTypeStr=uint8
  convert_in : FVT_lib/hal/convert_in  gain=0.1  offset=-6
  VHAL_ACCJerkLowerLimit_mps3 : Outport
  wires:
  convert_in/1 -> VHAL_ACCJerkLowerLimit_mps3/1
  UnitConverter/1 -> convert_in/1
  ACC_JerkLowerLimit/1 -> UnitConverter/1

== system halin/HAL_IN/CAN6/FCM1/ACCJerkUpperLimit ==
  ACC_JerkUpperLimit : Inport
  UnitConverter : DataTypeConversion  OutDataTypeStr=uint8
  convert_in : FVT_lib/hal/convert_in  gain=0.1  offset=-6
  VHAL_ACCJerkUpperLimit_mps3 : Outport
  wires:
  convert_in/1 -> VHAL_ACCJerkUpperLimit_mps3/1
  UnitConverter/1 -> convert_in/1
  ACC_JerkUpperLimit/1 -> UnitConverter/1

== system halin/HAL_IN/CAN6/FCM1/ACCObjDist ==
  ACC_ObjDist : Inport
  UnitConverter : DataTypeConversion  OutDataTypeStr=uint16
  convert_in : FVT_lib/hal/convert_in  gain=0.1  offset=0
  VHAL_ACCObjDist_m : Outport
  wires:
  convert_in/1 -> VHAL_ACCObjDist_m/1
  UnitConverter/1 -> convert_in/1
  ACC_ObjDist/1 -> UnitConverter/1

== system halin/HAL_IN/CAN6/FCM1/ACCObjDstLvl ==
  ACC_ObjDstLvl : Inport
  UnitConverter : DataTypeConversion  OutDataTypeStr=uint8
  VHAL_ACCObjDstLvl_enum : Outport
  wires:
  UnitConverter/1 -> VHAL_ACCObjDstLvl_enum/1
  ACC_ObjDstLvl/1 -> UnitConverter/1

== system halin/HAL_IN/CAN6/FCM1/ACCObjRelSpd ==
  ACC_ObjRelSpd : Inport
  UnitConverter : DataTypeConversion  OutDataTypeStr=uint16
  convert_in : FVT_lib/hal/convert_in  gain=0.1  offset=-100
  VHAL_ACCObjRelSpd_mps : Outport
  wires:
  convert_in/1 -> VHAL_ACCObjRelSpd_mps/1
  UnitConverter/1 -> convert_in/1
  ACC_ObjRelSpd/1 -> UnitConverter/1

== system halin/HAL_IN/CAN6/FCM1/ACCRequiredAccel ==
  ACC_RequiredAccel : Inport
  UnitConverter : DataTypeConversion  OutDataTypeStr=uint16
  convert_in : FVT_lib/hal/convert_in  gain=0.05  offset=-15
  VHAL_ACCRequiredAccel_mps2 : Outport
  wires:
  convert_in/1 -> VHAL_ACCRequiredAccel_mps2/1
  UnitConverter/1 -> convert_in/1
  ACC_RequiredAccel/1 -> UnitConverter/1

== system halin/HAL_IN/CAN6/FCM1/ACCTakeoverReq ==
  ACC_TakeoverReq : Inport
  UnitConverter : DataTypeConversion  OutDataTypeStr=uint8
  VHAL_ACCTakeoverReq_flg : Outport
  wires:
  UnitConverter/1 -> VHAL_ACCTakeoverReq_flg/1
  ACC_TakeoverReq/1 -> UnitConverter/1

== system halin/HAL_IN/CAN6/FCM1/ACCVehHoldReq ==
  ACC_VehHoldReq : Inport
  UnitConverter : DataTypeConversion  OutDataTypeStr=uint8
  VHAL_ACCVehHoldReq_flg : Outport
  wires:
  UnitConverter/1 -> VHAL_ACCVehHoldReq_flg/1
  ACC_VehHoldReq/1 -> UnitConverter/1

== system halin/HAL_IN/CAN6/FCM1/ADASACCSta ==
  ADAS_ACC_Sta : Inport
  UnitConverter : DataTypeConversion  OutDataTypeStr=uint8
  VHAL_ADASACCSta_enum : Outport
  wires:
  UnitConverter/1 -> VHAL_ADASACCSta_enum/1
  ADAS_ACC_Sta/1 -> UnitConverter/1

== system halin/HAL_IN/CAN6/FCM1/ADASAEBReq ==
  ADAS_AEBReq : Inport
  UnitConverter : DataTypeConversion  OutDataTypeStr=uint8
  VHAL_ADASAEBReq_enum : Outport
  wires:
  UnitConverter/1 -> VHAL_ADASAEBReq_enum/1
  ADAS_AEBReq/1 -> UnitConverter/1

== system halin/HAL_IN/CAN6/FCM1/ADASAEBSta ==
  ADAS_AEB_Sta : Inport
  UnitConverter : DataTypeConversion  OutDataTypeStr=uint8
  VHAL_ADASAEBSta_enum : Outport
  wires:
  UnitConverter/1 -> VHAL_ADASAEBSta_enum/1
  ADAS_AEB_Sta/1 -> UnitConverter/1

== system halin/HAL_IN/CAN6/FCM1/ADASCAMSpdLim ==
  ADAS_CAM_SpdLim : Inport
  UnitConverter : DataTypeConversion  OutDataTypeStr=uint8
  VHAL_ADASCAMSpdLim_enum : Outport
  wires:
  UnitConverter/1 -> VHAL_ADASCAMSpdLim_enum/1
  ADAS_CAM_SpdLim/1 -> UnitConverter/1

== system halin/HAL_IN/CAN6/FCM1/ADASDBSReq ==
  ADAS_DBSReq : Inport
  UnitConverter : DataTypeConversion  OutDataTypeStr=uint8
  VHAL_ADASDBSReq_enum : Outport
  wires:
  UnitConverter/1 -> VHAL_ADASDBSReq_enum/1
  ADAS_DBSReq/1 -> UnitConverter/1

== system halin/HAL_IN/CAN6/FCM1/ADASFCWMute ==
  ADAS_FCW_Mute : Inport
  UnitConverter : DataTypeConversion  OutDataTypeStr=uint8
  VHAL_ADASFCWMute_flg : Outport
  wires:
  UnitConverter/1 -> VHAL_ADASFCWMute_flg/1
  ADAS_FCW_Mute/1 -> UnitConverter/1

== system halin/HAL_IN/CAN6/FCM1/ADASFCWSta ==
  ADAS_FCW_Sta : Inport
  UnitConverter : DataTypeConversion  OutDataTypeStr=uint8
  VHAL_ADASFCWSta_enum : Outport
  wires:
  UnitConverter/1 -> VHAL_ADASFCWSta_enum/1
  ADAS_FCW_Sta/1 -> UnitConverter/1

== system halin/HAL_IN/CAN6/FCM1/ADASFaultSta ==
  ADAS_FaultSta : Inport
  UnitConverter : DataTypeConversion  OutDataTypeStr=uint8
  VHAL_ADASFaultSta_flg : Outport
  wires:
  UnitConverter/1 -> VHAL_ADASFaultSta_flg/1
  ADAS_FaultSta/1 -> UnitConverter/1

== system halin/HAL_IN/CAN6/FCM1/ADASFltWrnReq ==
  ADAS_FltWrnReq : Inport
  UnitConverter : DataTypeConversion  OutDataTypeStr=uint8
  VHAL_ADASFltWrnReq_flg : Outport
  wires:
  UnitConverter/1 -> VHAL_ADASFltWrnReq_flg/1
  ADAS_FltWrnReq/1 -> UnitConverter/1

== system halin/HAL_IN/CAN6/FCM1/ADASForceIdle ==
  ADAS_ForceIdle : Inport
  UnitConverter : DataTypeConversion  OutDataTypeStr=uint8
  VHAL_ADASForceIdle_flg : Outport
  wires:
  UnitConverter/1 -> VHAL_ADASForceIdle_flg/1
  ADAS_ForceIdle/1 -> UnitConverter/1

== system halin/HAL_IN/CAN6/FCM1/ADASISASta ==
  ADAS_ISA_Sta : Inport
  UnitConverter : DataTypeConversion  OutDataTypeStr=uint8
  VHAL_ADASISASta_enum : Outport
  wires:
  UnitConverter/1 -> VHAL_ADASISASta_enum/1
  ADAS_ISA_Sta/1 -> UnitConverter/1

== system halin/HAL_IN/CAN6/FCM1/ADASLDWMute ==
  ADAS_LDW_Mute : Inport
  UnitConverter : DataTypeConversion  OutDataTypeStr=uint8
  VHAL_ADASLDWMute_flg : Outport
  wires:
  UnitConverter/1 -> VHAL_ADASLDWMute_flg/1
  ADAS_LDW_Mute/1 -> UnitConverter/1

== system halin/HAL_IN/CAN6/FCM1/ADASLDWSta ==
  ADAS_LDW_Sta : Inport
  UnitConverter : DataTypeConversion  OutDataTypeStr=uint8
  VHAL_ADASLDWSta_enum : Outport
  wires:
  UnitConverter/1 -> VHAL_ADASLDWSta_enum/1
  ADAS_LDW_Sta/1 -> UnitConverter/1

== system halin/HAL_IN/CAN6/FCM1/ADASLFCHandsOffWarning ==
  ADAS_LFC_Hands_Off_Warning : Inport
  UnitConverter : DataTypeConversion  OutDataTypeStr=uint8
  VHAL_ADASLFCHandsOffWarning_enum : Outport
  wires:
  UnitConverter/1 -> VHAL_ADASLFCHandsOffWarning_enum/1
  ADAS_LFC_Hands_Off_Warning/1 -> UnitConverter/1

== system halin/HAL_IN/CAN6/FCM1/ADASLFCSta ==
  ADAS_LFC_Sta : Inport
  UnitConverter : DataTypeConversion  OutDataTypeStr=uint8
  VHAL_ADASLFCSta_enum : Outport
  wires:
  UnitConverter/1 -> VHAL_ADASLFCSta_enum/1
  ADAS_LFC_Sta/1 -> UnitConverter/1

== system halin/HAL_IN/CAN6/FCM1/ADASLFCWarnSound ==
  ADAS_LFC_Warn_Sound : Inport
  UnitConverter : DataTypeConversion  OutDataTypeStr=uint16
  VHAL_ADASLFCWarnSound_enum : Outport
  wires:
  UnitConverter/1 -> VHAL_ADASLFCWarnSound_enum/1
  ADAS_LFC_Warn_Sound/1 -> UnitConverter/1

== system halin/HAL_IN/CAN6/FCM1/ADASLKASta ==
  ADAS_LKA_Sta : Inport
  UnitConverter : DataTypeConversion  OutDataTypeStr=uint16
  VHAL_ADASLKASta_enum : Outport
  wires:
  UnitConverter/1 -> VHAL_ADASLKASta_enum/1
  ADAS_LKA_Sta/1 -> UnitConverter/1

== system halin/HAL_IN/CAN6/FCM1/ADASLaneModeL ==
  ADAS_LaneModeL : Inport
  UnitConverter : DataTypeConversion  OutDataTypeStr=uint16
  VHAL_ADASLaneModeL_enum : Outport
  wires:
  UnitConverter/1 -> VHAL_ADASLaneModeL_enum/1
  ADAS_LaneModeL/1 -> UnitConverter/1

== system halin/HAL_IN/CAN6/FCM1/ADASLaneModeR ==
  ADAS_LaneModeR : Inport
  UnitConverter : DataTypeConversion  OutDataTypeStr=uint8
  VHAL_ADASLaneModeR_enum : Outport
  wires:
  UnitConverter/1 -> VHAL_ADASLaneModeR_enum/1
  ADAS_LaneModeR/1 -> UnitConverter/1

== system halin/HAL_IN/CAN6/FCM1/ADASLanecurveL ==
  ADAS_Lane_curveL : Inport
  UnitConverter : DataTypeConversion  OutDataTypeStr=uint8
  convert_in : FVT_lib/hal/convert_in  gain=0.0005  offset=-0.03
  VHAL_ADASLanecurveL_raw32 : Outport
  wires:
  convert_in/1 -> VHAL_ADASLanecurveL_raw32/1
  UnitConverter/1 -> convert_in/1
  ADAS_Lane_curveL/1 -> UnitConverter/1

== system halin/HAL_IN/CAN6/FCM1/ADASLanecurveR ==
  ADAS_Lane_curveR : Inport
  UnitConverter : DataTypeConversion  OutDataTypeStr=uint8
  convert_in : FVT_lib/hal/convert_in  gain=0.0005  offset=-0.03
  VHAL_ADASLanecurveR_raw32 : Outport
  wires:
  convert_in/1 -> VHAL_ADASLanecurveR_raw32/1
  UnitConverter/1 -> convert_in/1
  ADAS_Lane_curveR/1 -> UnitConverter/1

== system halin/HAL_IN/CAN6/FCM1/ADASLanetypeL ==
  ADAS_LanetypeL : Inport
  UnitConverter : DataTypeConversion  OutDataTypeStr=uint16
  VHAL_ADASLanetypeL_enum : Outport
  wires:
  UnitConverter/1 -> VHAL_ADASLanetypeL_enum/1
  ADAS_LanetypeL/1 -> UnitConverter/1

== system halin/HAL_IN/CAN6/FCM1/ADASLanetypeR ==
  ADAS_LanetypeR : Inport
  UnitConverter : DataTypeConversion  OutDataTypeStr=uint8
  VHAL_ADASLanetypeR_enum : Outport
  wires:
  UnitConverter/1 -> VHAL_ADASLanetypeR_enum/1
  ADAS_LanetypeR/1 -> UnitConverter/1

== system halin/HAL_IN/CAN6/FCM1/ADASSLIFSpdLim ==
  ADAS_SLIF_SpdLim : Inport
  UnitConverter : DataTypeConversion  OutDataTypeStr=uint8
  VHAL_ADASSLIFSpdLim_enum : Outport
  wires:
  UnitConverter/1 -> VHAL_ADASSLIFSpdLim_enum/1
  ADAS_SLIF_SpdLim/1 -> UnitConverter/1

== system halin/HAL_IN/CAN6/FCM1/ADASSLIFSta ==
  ADAS_SLIF_Sta : Inport
  UnitConverter : DataTypeConversion  OutDataTypeStr=uint8
  VHAL_ADASSLIFSta_enum : Outport
  wires:
  UnitConverter/1 -> VHAL_ADASSLIFSta_enum/1
  ADAS_SLIF_Sta/1 -> UnitConverter/1

== system halin/HAL_IN/CAN6/FCM1/ADASShftPosnReq ==
  ADAS_ShftPosnReq : Inport
  UnitConverter : DataTypeConversion  OutDataTypeStr=uint8
  VHAL_ADASShftPosnReq_enum : Outport
  wires:
  UnitConverter/1 -> VHAL_ADASShftPosnReq_enum/1
  ADAS_ShftPosnReq/1 -> UnitConverter/1

== system halin/HAL_IN/CAN6/FCM1/ADASShftPosnReqA ==
  ADAS_ShftPosnReq_A : Inport
  UnitConverter : DataTypeConversion  OutDataTypeStr=uint8
  VHAL_ADASShftPosnReqA_flg : Outport
  wires:
  UnitConverter/1 -> VHAL_ADASShftPosnReqA_flg/1
  ADAS_ShftPosnReq_A/1 -> UnitConverter/1

== system halin/HAL_IN/CAN6/FCM1/ADASVehSpdLim ==
  ADAS_VehSpdLim : Inport
  UnitConverter : DataTypeConversion  OutDataTypeStr=uint8
  VHAL_ADASVehSpdLim_enum : Outport
  wires:
  UnitConverter/1 -> VHAL_ADASVehSpdLim_enum/1
  ADAS_VehSpdLim/1 -> UnitConverter/1

== system halin/HAL_IN/CAN6/FCM1/ADASWarningMsg ==
  ADAS_WarningMsg : Inport
  UnitConverter : DataTypeConversion  OutDataTypeStr=uint8
  VHAL_ADASWarningMsg_enum : Outport
  wires:
  UnitConverter/1 -> VHAL_ADASWarningMsg_enum/1
  ADAS_WarningMsg/1 -> UnitConverter/1

== system halin/HAL_IN/CAN6/FCM1/AEBVehHoldReq ==
  AEB_VehHoldReq : Inport
  UnitConverter : DataTypeConversion  OutDataTypeStr=uint8
  VHAL_AEBVehHoldReq_flg : Outport
  wires:
  UnitConverter/1 -> VHAL_AEBVehHoldReq_flg/1
  AEB_VehHoldReq/1 -> UnitConverter/1

== system halin/HAL_IN/CAN6/FCM1/CameraBlockage ==
  CameraBlockage : Inport
  UnitConverter : DataTypeConversion  OutDataTypeStr=uint8
  VHAL_CameraBlockage_flg : Outport
  wires:
  UnitConverter/1 -> VHAL_CameraBlockage_flg/1
  CameraBlockage/1 -> UnitConverter/1

== system halin/HAL_IN/CAN6/FCM1/FCM1Checksum ==
  FCM1_Checksum : Inport
  UnitConverter : DataTypeConversion  OutDataTypeStr=uint8
  VHAL_FCM1Checksum_enum : Outport
  wires:
  UnitConverter/1 -> VHAL_FCM1Checksum_enum/1
  FCM1_Checksum/1 -> UnitConverter/1

== system halin/HAL_IN/CAN6/FCM1/FCM1LifeCount ==
  FCM1_LifeCount : Inport
  UnitConverter : DataTypeConversion  OutDataTypeStr=uint8
  VHAL_FCM1LifeCount_enum : Outport
  wires:
  UnitConverter/1 -> VHAL_FCM1LifeCount_enum/1
  FCM1_LifeCount/1 -> UnitConverter/1

== system halin/HAL_IN/CAN6/FCM1/FCMACCmode ==
  FCM_ACCmode : Inport
  UnitConverter : DataTypeConversion  OutDataTypeStr=uint8
  VHAL_FCMACCmode_enum : Outport
  wires:
  UnitConverter/1 -> VHAL_FCMACCmode_enum/1
  FCM_ACCmode/1 -> UnitConverter/1

== system halin/HAL_IN/CAN6/FCM1/FCMLKAStrToqReq ==
  FCM_LKA_StrToqReq : Inport
  UnitConverter : DataTypeConversion  OutDataTypeStr=uint16
  convert_in : FVT_lib/hal/convert_in  gain=0.008  offset=-8
  VHAL_FCMLKAStrToqReq_Nm : Outport
  wires:
  convert_in/1 -> VHAL_FCMLKAStrToqReq_Nm/1
  UnitConverter/1 -> convert_in/1
  FCM_LKA_StrToqReq/1 -> UnitConverter/1

== system halin/HAL_IN/CAN6/FCM1/FCMLKATOIAct ==
  FCM_LKA_TOIAct : Inport
  UnitConverter : DataTypeConversion  OutDataTypeStr=uint8
  VHAL_FCMLKATOIAct_enum : Outport
  wires:
  UnitConverter/1 -> VHAL_FCMLKATOIAct_enum/1
  FCM_LKA_TOIAct/1 -> UnitConverter/1

== system halin/HAL_IN/CAN6/FCM1/FCMLKATOIFault ==
  FCM_LKA_TOIFault : Inport
  UnitConverter : DataTypeConversion  OutDataTypeStr=uint8
  VHAL_FCMLKATOIFault_flg : Outport
  wires:
  UnitConverter/1 -> VHAL_FCMLKATOIFault_flg/1
  FCM_LKA_TOIFault/1 -> UnitConverter/1

== system halin/HAL_IN/CAN6/FCM1/ForceLowBeam ==
  ForceLowBeam : Inport
  UnitConverter : DataTypeConversion  OutDataTypeStr=uint8
  VHAL_ForceLowBeam_enum : Outport
  wires:
  UnitConverter/1 -> VHAL_ForceLowBeam_enum/1
  ForceLowBeam/1 -> UnitConverter/1

== system halin/HAL_IN/CAN6/FCM1/HazardWarningReq ==
  HazardWarningReq : Inport
  UnitConverter : DataTypeConversion  OutDataTypeStr=uint8
  VHAL_HazardWarningReq_flg : Outport
  wires:
  UnitConverter/1 -> VHAL_HazardWarningReq_flg/1
  HazardWarningReq/1 -> UnitConverter/1

== system halin/HAL_IN/CAN6/FCM1/ISAWarningMsg ==
  ISA_WarningMsg : Inport
  UnitConverter : DataTypeConversion  OutDataTypeStr=uint8
  VHAL_ISAWarningMsg_enum : Outport
  wires:
  UnitConverter/1 -> VHAL_ISAWarningMsg_enum/1
  ISA_WarningMsg/1 -> UnitConverter/1

== system halin/HAL_IN/CAN6/FCM1/LKAHODDisplayWarning ==
  LKA_HOD_Display_Warning : Inport
  UnitConverter : DataTypeConversion  OutDataTypeStr=uint8
  VHAL_LKAHODDisplayWarning_flg : Outport
  wires:
  UnitConverter/1 -> VHAL_LKAHODDisplayWarning_flg/1
  LKA_HOD_Display_Warning/1 -> UnitConverter/1

== system halin/HAL_IN/CAN6/FCM1/LKAHODSoundWarning ==
  LKA_HOD_Sound_Warning : Inport
  UnitConverter : DataTypeConversion  OutDataTypeStr=uint8
  VHAL_LKAHODSoundWarning_flg : Outport
  wires:
  UnitConverter/1 -> VHAL_LKAHODSoundWarning_flg/1
  LKA_HOD_Sound_Warning/1 -> UnitConverter/1

== system halin/HAL_IN/CAN6/FCM1/LVDAACCStatusInformation ==
  LVDA_ACCStatusInformation : Inport
  UnitConverter : DataTypeConversion  OutDataTypeStr=uint8
  VHAL_LVDAACCStatusInformation_flg : Outport
  wires:
  UnitConverter/1 -> VHAL_LVDAACCStatusInformation_flg/1
  LVDA_ACCStatusInformation/1 -> UnitConverter/1

== system halin/HAL_IN/CAN6/FCM1/LVDADisabled ==
  LVDA_Disabled : Inport
  UnitConverter : DataTypeConversion  OutDataTypeStr=uint8
  VHAL_LVDADisabled_flg : Outport
  wires:
  UnitConverter/1 -> VHAL_LVDADisabled_flg/1
  LVDA_Disabled/1 -> UnitConverter/1

== system halin/HAL_IN/CAN6/FCM1/LVDAFailinfo ==
  LVDA_Failinfo : Inport
  UnitConverter : DataTypeConversion  OutDataTypeStr=uint8
  VHAL_LVDAFailinfo_flg : Outport
  wires:
  UnitConverter/1 -> VHAL_LVDAFailinfo_flg/1
  LVDA_Failinfo/1 -> UnitConverter/1

== system halin/HAL_IN/CAN6/FCM1/LVDAMuteSta ==
  LVDA_Mute_Sta : Inport
  UnitConverter : DataTypeConversion  OutDataTypeStr=uint8
  VHAL_LVDAMuteSta_enum : Outport
  wires:
  UnitConverter/1 -> VHAL_LVDAMuteSta_enum/1
  LVDA_Mute_Sta/1 -> UnitConverter/1

== system halin/HAL_IN/CAN6/FCM1/LVDAWarning ==
  LVDA_Warning : Inport
  UnitConverter : DataTypeConversion  OutDataTypeStr=uint8
  VHAL_LVDAWarning_flg : Outport
  wires:
  UnitConverter/1 -> VHAL_LVDAWarning_flg/1
  LVDA_Warning/1 -> UnitConverter/1

== system halin/HAL_IN/CAN6/FCM1/LeftTurnLightReq ==
  LeftTurnLightReq : Inport
  UnitConverter : DataTypeConversion  OutDataTypeStr=uint8
  VHAL_LeftTurnLightReq_flg : Outport
  wires:
  UnitConverter/1 -> VHAL_LeftTurnLightReq_flg/1
  LeftTurnLightReq/1 -> UnitConverter/1

== system halin/HAL_IN/CAN6/FCM1/RightTurnLightReq ==
  RightTurnLightReq : Inport
  UnitConverter : DataTypeConversion  OutDataTypeStr=uint8
  VHAL_RightTurnLightReq_flg : Outport
  wires:
  UnitConverter/1 -> VHAL_RightTurnLightReq_flg/1
  RightTurnLightReq/1 -> UnitConverter/1

== system halin/HAL_IN/CAN6/FCM1/TargetType ==
  Target_Type : Inport
  UnitConverter : DataTypeConversion  OutDataTypeStr=uint16
  VHAL_TargetType_enum : Outport
  wires:
  UnitConverter/1 -> VHAL_TargetType_enum/1
  Target_Type/1 -> UnitConverter/1

== system halin/HAL_IN/CAN6/FCM1/TimeGapLevel ==
  TimeGapLevel : Inport
  UnitConverter : DataTypeConversion  OutDataTypeStr=uint8
  VHAL_TimeGapLevel_enum : Outport
  wires:
  UnitConverter/1 -> VHAL_TimeGapLevel_enum/1
  TimeGapLevel/1 -> UnitConverter/1

== system halin/HAL_IN/CAN6/FCM2/ADBVehDst1Val ==
  ADB_VehDst1Val : Inport
  UnitConverter : DataTypeConversion  OutDataTypeStr=uint8
  VHAL_ADBVehDst1Val_enum : Outport
  wires:
  UnitConverter/1 -> VHAL_ADBVehDst1Val_enum/1
  ADB_VehDst1Val/1 -> UnitConverter/1

== system halin/HAL_IN/CAN6/FCM3/MELaneCurvDervLt ==
  ME_Lane_CurvDervLt : Inport
  UnitConverter : DataTypeConversion  OutDataTypeStr=uint16
  convert_in : FVT_lib/hal/convert_in  gain=4e-09  offset=-0.00013
  VHAL_MELaneCurvDervLt_raw32 : Outport
  wires:
  convert_in/1 -> VHAL_MELaneCurvDervLt_raw32/1
  UnitConverter/1 -> convert_in/1
  ME_Lane_CurvDervLt/1 -> UnitConverter/1

== system halin/HAL_IN/CAN6/FCM3/MELaneCurvDervLt2 ==
  ME_Lane_CurvDervLt2 : Inport
  UnitConverter : DataTypeConversion  OutDataTypeStr=uint16
  convert_in : FVT_lib/hal/convert_in  gain=4e-09  offset=-0.00013
  VHAL_MELaneCurvDervLt2_raw32 : Outport
  wires:
  convert_in/1 -> VHAL_MELaneCurvDervLt2_raw32/1
  UnitConverter/1 -> convert_in/1
  ME_Lane_CurvDervLt2/1 -> UnitConverter/1

== system halin/HAL_IN/CAN6/FCM3/MELaneCurvDervRt ==
  ME_Lane_CurvDervRt : Inport
  UnitConverter : DataTypeConversion  OutDataTypeStr=uint16
  convert_in : FVT_lib/hal/convert_in  gain=4e-09  offset=-0.00013
  VHAL_MELaneCurvDervRt_raw32 : Outport
  wires:
  convert_in/1 -> VHAL_MELaneCurvDervRt_raw32/1
  UnitConverter/1 -> convert_in/1
  ME_Lane_CurvDervRt/1 -> UnitConverter/1

== system halin/HAL_IN/CAN6/FCM3/MELaneCurvDervRt2 ==
  ME_Lane_CurvDervRt2 : Inport
  UnitConverter : DataTypeConversion  OutDataTypeStr=uint16
  convert_in : FVT_lib/hal/convert_in  gain=4e-09  offset=-0.00013
  VHAL_MELaneCurvDervRt2_raw32 : Outport
  wires:
  convert_in/1 -> VHAL_MELaneCurvDervRt2_raw32/1
  UnitConverter/1 -> convert_in/1
  ME_Lane_CurvDervRt2/1 -> UnitConverter/1

== system halin/HAL_IN/CAN6/FCM3/MELaneCurvLt ==
  ME_Lane_CurvLt : Inport
  UnitConverter : DataTypeConversion  OutDataTypeStr=uint16
  convert_in : FVT_lib/hal/convert_in  gain=1e-06  offset=-0.032
  VHAL_MELaneCurvLt_raw32 : Outport
  wires:
  convert_in/1 -> VHAL_MELaneCurvLt_raw32/1
  UnitConverter/1 -> convert_in/1
  ME_Lane_CurvLt/1 -> UnitConverter/1

== system halin/HAL_IN/CAN6/FCM3/MELaneCurvLt2 ==
  ME_Lane_CurvLt2 : Inport
  UnitConverter : DataTypeConversion  OutDataTypeStr=uint16
  convert_in : FVT_lib/hal/convert_in  gain=1e-06  offset=-0.032
  VHAL_MELaneCurvLt2_raw32 : Outport
  wires:
  convert_in/1 -> VHAL_MELaneCurvLt2_raw32/1
  UnitConverter/1 -> convert_in/1
  ME_Lane_CurvLt2/1 -> UnitConverter/1

== system halin/HAL_IN/CAN6/FCM3/MELaneCurvRt ==
  ME_Lane_CurvRt : Inport
  UnitConverter : DataTypeConversion  OutDataTypeStr=uint16
  convert_in : FVT_lib/hal/convert_in  gain=1e-06  offset=-0.032
  VHAL_MELaneCurvRt_raw32 : Outport
  wires:
  convert_in/1 -> VHAL_MELaneCurvRt_raw32/1
  UnitConverter/1 -> convert_in/1
  ME_Lane_CurvRt/1 -> UnitConverter/1

== system halin/HAL_IN/CAN6/FCM3/MELaneCurvRt2 ==
  ME_Lane_CurvRt2 : Inport
  UnitConverter : DataTypeConversion  OutDataTypeStr=uint16
  convert_in : FVT_lib/hal/convert_in  gain=1e-06  offset=-0.032
  VHAL_MELaneCurvRt2_raw32 : Outport
  wires:
  convert_in/1 -> VHAL_MELaneCurvRt2_raw32/1
  UnitConverter/1 -> convert_in/1
  ME_Lane_CurvRt2/1 -> UnitConverter/1

== system halin/HAL_IN/CAN6/FCM3/MELaneHeadAngLt ==
  ME_Lane_HeadAngLt : Inport
  UnitConverter : DataTypeConversion  OutDataTypeStr=uint16
  convert_in : FVT_lib/hal/convert_in  gain=0.001  offset=-0.5
  VHAL_MELaneHeadAngLt_radians : Outport
  wires:
  convert_in/1 -> VHAL_MELaneHeadAngLt_radians/1
  UnitConverter/1 -> convert_in/1
  ME_Lane_HeadAngLt/1 -> UnitConverter/1

== system halin/HAL_IN/CAN6/FCM3/MELaneHeadAngLt2 ==
  ME_Lane_HeadAngLt2 : Inport
  UnitConverter : DataTypeConversion  OutDataTypeStr=uint16
  convert_in : FVT_lib/hal/convert_in  gain=0.001  offset=-0.5
  VHAL_MELaneHeadAngLt2_radians : Outport
  wires:
  convert_in/1 -> VHAL_MELaneHeadAngLt2_radians/1
  UnitConverter/1 -> convert_in/1
  ME_Lane_HeadAngLt2/1 -> UnitConverter/1
